simulink model "BalRobModel"  (R2021a)
settings: Solver=FixedStepAuto  StartTime=0.0  StopTime=20  FixedStep=Ts  RelTol=1e-3
undefined symbols (not defined in the file): body, DiscIntNeverNeededParam, drv, g, gbox, lqr_nominal, lqr_robust, mot, ms22g, nlmodel, Nu, Nx, sens, stvar_est, Ts, wheel
settings Model: Creator=gioel  LastModifiedBy=gioel
settings DataIOCC: LimitDataPoints=on  MaxDataPoints=50000  ReturnWorkspaceOutputs=off
settings DebuggingCC: AlgebraicLoopMsg=none

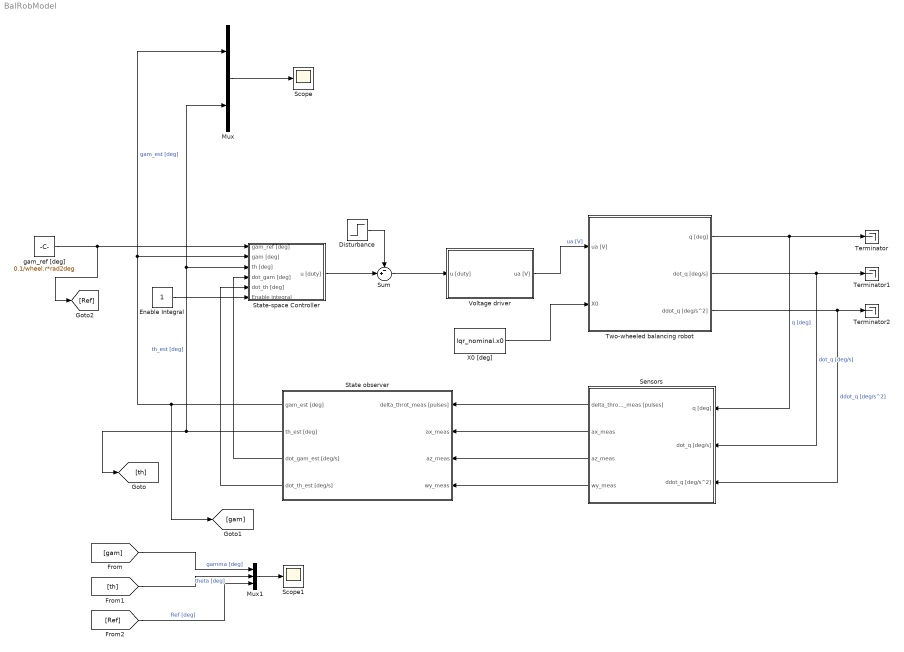
== system BalRobModel ==
  Disturbance : Step  Time=10  After=5/drv.duty2V  SampleTime=0
  Enable Integral : Constant
  Mux : Mux  Inputs=2
  Mux1 : Mux  Inputs=3
  Scope : Scope
  Scope1 : Scope
  Sensors : Subsystem
  State observer : Subsystem
  State-space Controller : Subsystem
  Sum : Sum  Inputs=-+|
  Terminator : Terminator
  Terminator1 : Terminator
  Terminator2 : Terminator
  Two-wheeled balancing robot : Subsystem
  Voltage driver : Subsystem
  X0 [deg] : Constant  Value=lqr_nominal.x0
  gam_ref [deg] : Constant  Value=0.1/wheel.r*rad2deg
  wires:
  Voltage driver/1(ua [V]) -> Two-wheeled balancing robot/1(ua [V])  "ua [V]"
  Two-wheeled balancing robot/1(q [deg]) -> Sensors/1(q [deg]), Terminator/1  "q [deg]"
  Two-wheeled balancing robot/2(dot_q [deg/s]) -> Sensors/2(dot_q [deg/s]), Terminator1/1  "dot_q [deg/s]"
  Two-wheeled balancing robot/3(ddot_q [deg/s^2]) -> Sensors/3(ddot_q [deg/s^2]), Terminator2/1  "ddot_q [deg/s^2]"
  State observer/2(th_est [deg]) -> [th], Mux/2, State-space Controller/3(th [deg])  "th_est [deg]"
  State observer/1(gam_est [deg]) -> [gam], Mux/1, State-space Controller/2(gam [deg])  "gam_est [deg]"
  State observer/3(dot_gam_est [deg/s]) -> State-space Controller/4(dot_gam [deg])
  Sensors/1(delta_throt_meas [pulses]) -> State observer/1(delta_throt_meas [pulses])
  Sensors/2(ax_meas) -> State observer/2(ax_meas)
  Sensors/3(az_meas) -> State observer/3(az_meas)
  Sensors/4(wy_meas) -> State observer/4(wy_meas)
  gam_ref [deg]/1 -> [Ref], State-space Controller/1(gam_ref [deg])
  State observer/4(dot_th_est [deg/s]) -> State-space Controller/5(dot_th [deg])
  Mux/1 -> Scope/1
  Enable Integral/1 -> State-space Controller/6(Enable integral)
  State-space Controller/1(u [duty]) -> Sum/2
  Sum/1 -> Voltage driver/1(u [duty])
  Disturbance/1 -> Sum/1
  X0 [deg]/1 -> Two-wheeled balancing robot/2(X0)
  [gam] -> Mux1/1  "gamma [deg]"
  [th] -> Mux1/2  "theta [deg]"
  Mux1/1 -> Scope1/1
  [Ref] -> Mux1/3  "Ref [deg]"

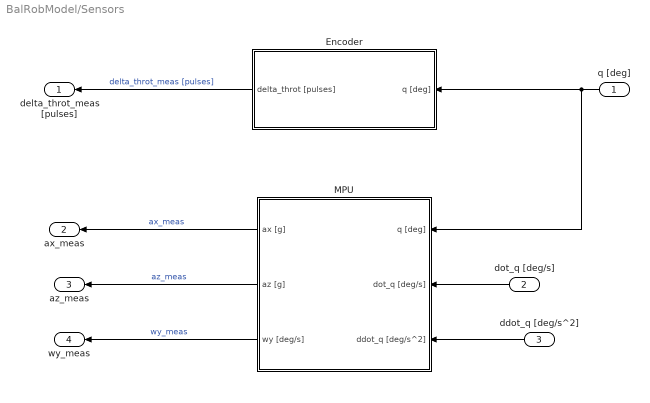
== system BalRobModel/Sensors ==
  q [deg] : Inport
  dot_q [deg/s] : Inport  Port=2
  ddot_q [deg/s^2] : Inport  Port=3
  Encoder : Subsystem
  MPU : Subsystem
  delta_throt_meas [pulses] : Outport
  ax_meas : Outport  Port=2
  az_meas : Outport  Port=3
  wy_meas : Outport  Port=4
  wires:
  Encoder/1(delta_throt [pulses]) -> delta_throt_meas [pulses]/1  "delta_throt_meas [pulses]"
  MPU/3(wy [deg/s]) -> wy_meas/1  "wy_meas"
  ddot_q [deg/s^2]/1 -> MPU/3(ddot_q [deg/s^2])
  MPU/2(az [g]) -> az_meas/1  "az_meas"
  dot_q [deg/s]/1 -> MPU/2(dot_q [deg/s])
  MPU/1(ax [g]) -> ax_meas/1  "ax_meas"
  q [deg]/1 -> MPU/1(q [deg]), Encoder/1(q [deg])

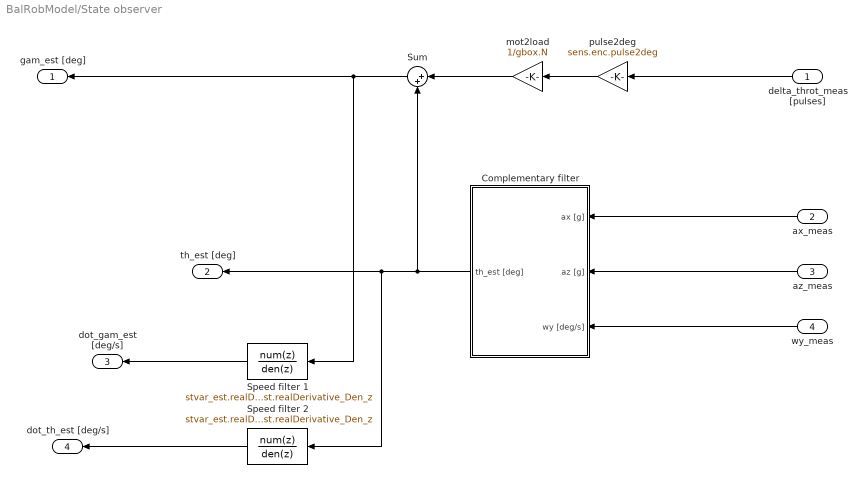
== system BalRobModel/State observer ==
  delta_throt_meas [pulses] : Inport
  ax_meas : Inport  Port=2
  az_meas : Inport  Port=3
  wy_meas : Inport  Port=4
  Complementary filter : Subsystem
  Speed filter 1 : DiscreteTransferFcn  Numerator=stvar_est.realDerivative_Num_z  Denominator=stvar_est.realDerivative_Den_z  SampleTime=Ts
  Speed filter 2 : DiscreteTransferFcn  Numerator=stvar_est.realDerivative_Num_z  Denominator=stvar_est.realDerivative_Den_z  SampleTime=Ts
  Sum : Sum  Inputs=|++
  mot2load : Gain  Gain=1/gbox.N
  pulse2deg : Gain  Gain=sens.enc.pulse2deg
  gam_est [deg] : Outport
  th_est [deg] : Outport  Port=2
  dot_gam_est [deg/s] : Outport  Port=3
  dot_th_est [deg/s] : Outport  Port=4
  wires:
  az_meas/1 -> Complementary filter/2(az [g])
  Speed filter 1/1 -> dot_gam_est [deg/s]/1
  Speed filter 2/1 -> dot_th_est [deg/s]/1
  wy_meas/1 -> Complementary filter/3(wy [deg/s])
  ax_meas/1 -> Complementary filter/1(ax [g])
  delta_throt_meas [pulses]/1 -> pulse2deg/1
  pulse2deg/1 -> mot2load/1
  mot2load/1 -> Sum/1
  Sum/1 -> gam_est [deg]/1, Speed filter 1/1
  Complementary filter/1(th_est [deg]) -> Sum/2, th_est [deg]/1, Speed filter 2/1

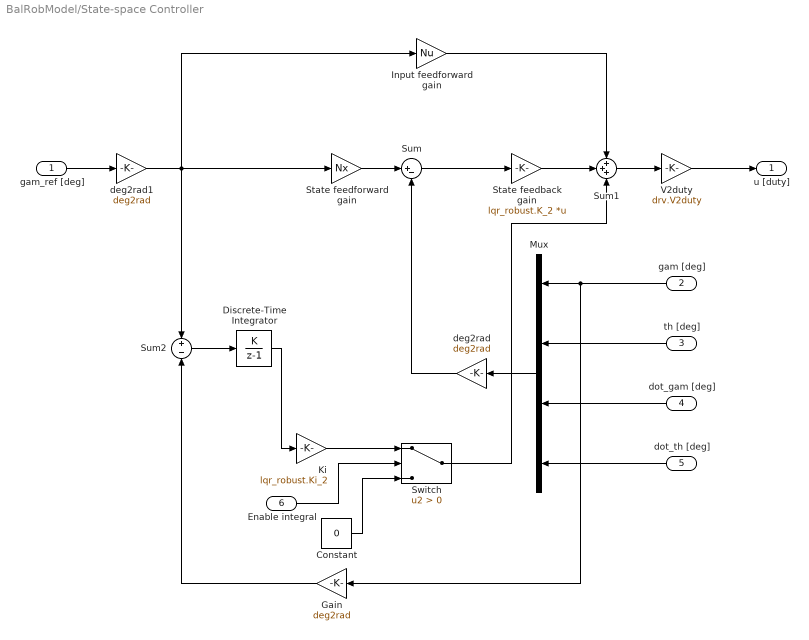
== system BalRobModel/State-space Controller ==
  gam_ref [deg] : Inport
  gam [deg] : Inport  Port=2
  th [deg] : Inport  Port=3
  dot_gam [deg] : Inport  Port=4
  dot_th [deg] : Inport  Port=5
  Enable integral : Inport  Port=6
  Constant : Constant  Value=0
  Discrete-Time Integrator : DiscreteIntegrator  IntegratorMethod=Accumulation: Forward Euler  SampleTime=Ts  ICPrevOutput=DiscIntNeverNeededParam  ICPrevScaledInput=DiscIntNeverNeededParam
  Gain : Gain  Gain=deg2rad
  Input feedforward gain : Gain  Gain=Nu
  Ki : Gain  Gain=lqr_robust.Ki_2
  Mux : Mux
  State feedback gain : Gain  Gain=lqr_robust.K_2  Multiplication=Matrix(K*u)
  State feedforward gain : Gain  Gain=Nx
  Sum : Sum  Inputs=|+-
  Sum1 : Sum  Inputs=+++
  Sum2 : Sum  Inputs=+|-
  Switch : Switch  Criteria=u2 > Threshold
  V2duty : Gain  Gain=drv.V2duty
  deg2rad : Gain  Gain=deg2rad
  deg2rad1 : Gain  Gain=deg2rad
  u [duty] : Outport
  wires:
  gam [deg]/1 -> Gain/1, Mux/1
  th [deg]/1 -> Mux/2
  dot_gam [deg]/1 -> Mux/3
  dot_th [deg]/1 -> Mux/4
  Mux/1 -> deg2rad/1
  gam_ref [deg]/1 -> deg2rad1/1
  deg2rad1/1 -> State feedforward gain/1, Input feedforward gain/1, Sum2/1
  State feedforward gain/1 -> Sum/1
  deg2rad/1 -> Sum/2
  Sum/1 -> State feedback gain/1
  State feedback gain/1 -> Sum1/2
  Input feedforward gain/1 -> Sum1/1
  Sum1/1 -> V2duty/1
  V2duty/1 -> u [duty]/1
  Gain/1 -> Sum2/2
  Sum2/1 -> Discrete-Time Integrator/1
  Discrete-Time Integrator/1 -> Ki/1
  Ki/1 -> Switch/1
  Switch/1 -> Sum1/3
  Enable integral/1 -> Switch/2
  Constant/1 -> Switch/3

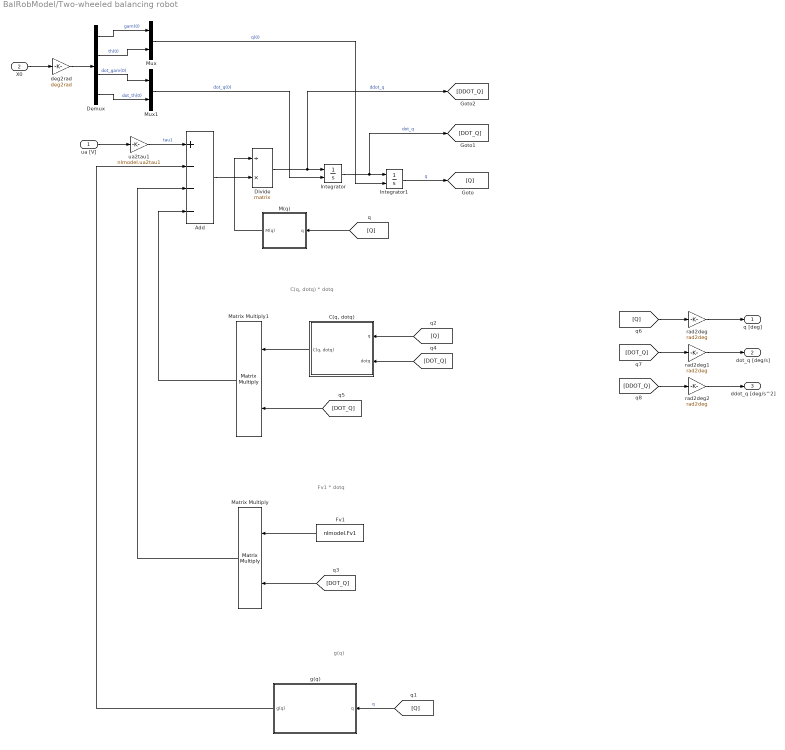
== system BalRobModel/Two-wheeled balancing robot ==
  note: g(q)
  note: Fv1 * dotq
  note: C(q, dotq) * dotq
  ua [V] : Inport
  X0 : Inport  Port=2
  Add : Sum  Inputs=+---
  "C(q, dotq)" : Subsystem
  Demux : Demux
  Divide : Product  Inputs=/*  Multiplication=Matrix(*)
  Fv1 : Constant  Value=nlmodel.Fv1
  Integrator : Integrator  InitialConditionSource=external  InitialCondition=[0;0]
  Integrator1 : Integrator  InitialConditionSource=external  InitialCondition=[0; 0]
  M(q) : Subsystem
  Matrix Multiply : Product  Multiplication=Matrix(*)
  Matrix Multiply1 : Product  Multiplication=Matrix(*)
  Mux : Mux  Inputs=2
  Mux1 : Mux  Inputs=2
  deg2rad : Gain  Gain=deg2rad
  g(q) : Subsystem
  rad2deg : Gain  Gain=rad2deg
  rad2deg1 : Gain  Gain=rad2deg
  rad2deg2 : Gain  Gain=rad2deg
  ua2tau1 : Gain  Gain=nlmodel.ua2tau1
  q [deg] : Outport
  dot_q [deg/s] : Outport  Port=2
  ddot_q [deg/s^2] : Outport  Port=3
  wires:
  [Q] -> M(q)/1(q)
  [Q] -> g(q)/1(q)  "q"
  [DOT_Q] -> rad2deg1/1
  rad2deg1/1 -> dot_q [deg/s]/1
  Matrix Multiply/1 -> Add/3
  Add/1 -> Divide/2
  Divide/1 -> [DDOT_Q], Integrator/1  "ddot_q"
  "C(q, dotq)"/1("C(q, dotq)") -> Matrix Multiply1/1
  rad2deg2/1 -> ddot_q [deg/s^2]/1
  g(q)/1(g(q)) -> Add/2
  M(q)/1(M(q)) -> Divide/1
  [Q] -> rad2deg/1
  [DDOT_Q] -> rad2deg2/1
  ua [V]/1 -> ua2tau1/1
  [Q] -> "C(q, dotq)"/1(q)
  Integrator/1 -> Integrator1/1, [DOT_Q]  "dot_q"
  ua2tau1/1 -> Add/1  "tau1"
  [DOT_Q] -> "C(q, dotq)"/2(dotq)
  [DOT_Q] -> Matrix Multiply/2
  [DOT_Q] -> Matrix Multiply1/2
  Integrator1/1 -> [Q]  "q"
  Matrix Multiply1/1 -> Add/4
  rad2deg/1 -> q [deg]/1
  Fv1/1 -> Matrix Multiply/1
  Demux/1 -> Mux/1  "gam(0)"
  Demux/2 -> Mux/2  "th(0)"
  Demux/3 -> Mux1/1  "dot_gam(0)"
  Demux/4 -> Mux1/2  "dot_th(0)"
  X0/1 -> deg2rad/1
  deg2rad/1 -> Demux/1
  Mux/1 -> Integrator1/2  "q(0)"
  Mux1/1 -> Integrator/2  "dot_q(0)"

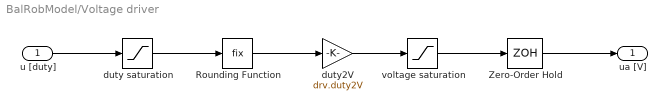
== system BalRobModel/Voltage driver ==
  u [duty] : Inport
  Rounding Function : Rounding  Operator=fix
  Zero-Order Hold : ZeroOrderHold  SampleTime=Ts
  duty saturation : Saturate  UpperLimit=drv.dutymax  LowerLimit=-drv.dutymax
  duty2V : Gain  Gain=drv.duty2V
  voltage saturation : Saturate  UpperLimit=drv.Vbus  LowerLimit=-drv.Vbus
  ua [V] : Outport
  wires:
  u [duty]/1 -> duty saturation/1
  duty saturation/1 -> Rounding Function/1
  Rounding Function/1 -> duty2V/1
  duty2V/1 -> voltage saturation/1
  voltage saturation/1 -> Zero-Order Hold/1
  Zero-Order Hold/1 -> ua [V]/1

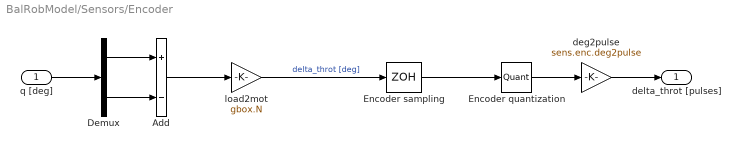
== system BalRobModel/Sensors/Encoder ==
  q [deg] : Inport
  Add : Sum  Inputs=+-
  Demux : Demux  Outputs=2
  Encoder quantization : Quantizer  QuantizationInterval=sens.enc.pulse2deg
  Encoder sampling : ZeroOrderHold  SampleTime=Ts
  deg2pulse : Gain  Gain=sens.enc.deg2pulse
  load2mot : Gain  Gain=gbox.N
  delta_throt [pulses] : Outport
  wires:
  q [deg]/1 -> Demux/1
  Demux/2 -> Add/2
  Demux/1 -> Add/1
  Add/1 -> load2mot/1
  load2mot/1 -> Encoder sampling/1  "delta_throt [deg]"
  Encoder sampling/1 -> Encoder quantization/1
  deg2pulse/1 -> delta_throt [pulses]/1
  Encoder quantization/1 -> deg2pulse/1

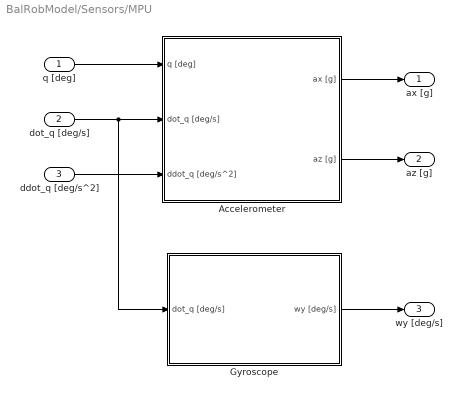
== system BalRobModel/Sensors/MPU ==
  q [deg] : Inport
  dot_q [deg/s] : Inport  Port=2
  ddot_q [deg/s^2] : Inport  Port=3
  "\tGyroscope" : Subsystem
  Accelerometer : Subsystem
  ax [g] : Outport
  az [g] : Outport  Port=2
  wy [deg/s] : Outport  Port=3
  wires:
  ddot_q [deg/s^2]/1 -> Accelerometer/3(ddot_q [deg/s^2])
  dot_q [deg/s]/1 -> "\tGyroscope"/1(dot_q [deg/s]), Accelerometer/2(dot_q [deg/s])
  q [deg]/1 -> Accelerometer/1(q [deg])
  "\tGyroscope"/1(wy [deg/s]) -> wy [deg/s]/1
  Accelerometer/2(az [g]) -> az [g]/1
  Accelerometer/1(ax [g]) -> ax [g]/1

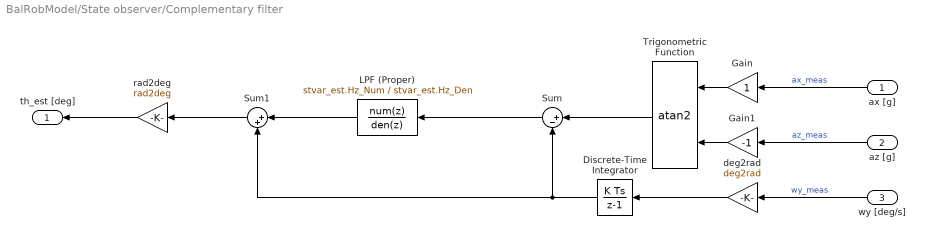
== system BalRobModel/State observer/Complementary filter ==
  ax [g] : Inport
  az [g] : Inport  Port=2
  wy [deg/s] : Inport  Port=3
  Discrete-Time Integrator : DiscreteIntegrator  SampleTime=Ts  ICPrevOutput=DiscIntNeverNeededParam  ICPrevScaledInput=DiscIntNeverNeededParam
  Gain : Gain
  Gain1 : Gain  Gain=-1
  LPF (Proper) : DiscreteTransferFcn  Numerator=stvar_est.Hz_Num  Denominator=stvar_est.Hz_Den  SampleTime=Ts
  Sum : Sum  Inputs=|+-
  Sum1 : Sum  Inputs=|++
  Trigonometric Function : Trigonometry  Operator=atan2
  deg2rad : Gain  Gain=deg2rad
  rad2deg : Gain  Gain=rad2deg
  th_est [deg] : Outport
  wires:
  LPF (Proper)/1 -> Sum1/1
  rad2deg/1 -> th_est [deg]/1
  Sum/1 -> LPF (Proper)/1
  Sum1/1 -> rad2deg/1
  Discrete-Time Integrator/1 -> Sum1/2, Sum/2
  Trigonometric Function/1 -> Sum/1
  wy [deg/s]/1 -> deg2rad/1  "wy_meas"
  az [g]/1 -> Gain1/1  "az_meas"
  ax [g]/1 -> Gain/1  "ax_meas"
  deg2rad/1 -> Discrete-Time Integrator/1
  Gain1/1 -> Trigonometric Function/2
  Gain/1 -> Trigonometric Function/1

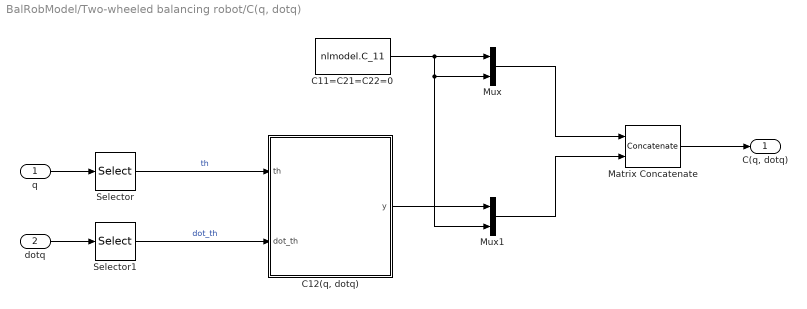
== system BalRobModel/Two-wheeled balancing robot/C(q, dotq) ==
  q : Inport
  dotq : Inport  Port=2
  C11=C21=C22=0 : Constant  Value=nlmodel.C_11
  "C12(q, dotq)" : MATLAB Function  TreatAsAtomicUnit=on
  Matrix Concatenate : Concatenate  Mode=Multidimensional array  ConcatenateDimension=2
  Mux : Mux  Inputs=2
  Mux1 : Mux  Inputs=2
  Selector : Selector  InputPortWidth=2  IndexOptions=Starting index (dialog)  Indices=2  OutputSizes=1
  Selector1 : Selector  InputPortWidth=2  IndexOptions=Starting index (dialog)  Indices=2  OutputSizes=1
  "C(q, dotq)" : Outport
  wires:
  Matrix Concatenate/1 -> "C(q, dotq)"/1
  "C12(q, dotq)"/1(y) -> Mux1/1
  q/1 -> Selector/1
  dotq/1 -> Selector1/1
  Selector1/1 -> "C12(q, dotq)"/2(dot_th)  "dot_th"
  Selector/1 -> "C12(q, dotq)"/1(th)  "th"
  C11=C21=C22=0/1 -> Mux/2, Mux1/2, Mux/1
  Mux/1 -> Matrix Concatenate/1
  Mux1/1 -> Matrix Concatenate/2

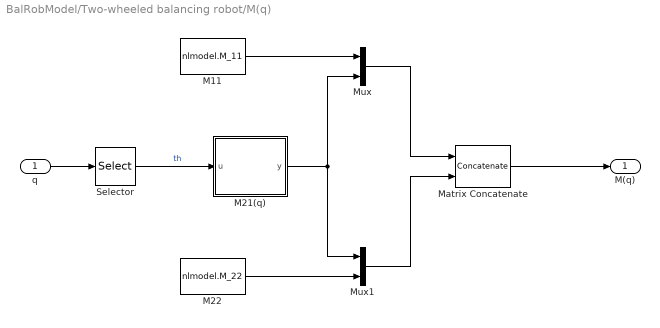
== system BalRobModel/Two-wheeled balancing robot/M(q) ==
  q : Inport
  M11 : Constant  Value=nlmodel.M_11
  M21(q) : MATLAB Function  TreatAsAtomicUnit=on
  M22 : Constant  Value=nlmodel.M_22
  Matrix Concatenate : Concatenate  Mode=Multidimensional array  ConcatenateDimension=2
  Mux : Mux  Inputs=2
  Mux1 : Mux  Inputs=2
  Selector : Selector  InputPortWidth=2  IndexOptions=Starting index (dialog)  Indices=2  OutputSizes=1
  M(q) : Outport
  wires:
  Matrix Concatenate/1 -> M(q)/1
  Mux1/1 -> Matrix Concatenate/2
  M22/1 -> Mux1/2
  M11/1 -> Mux/1
  Selector/1 -> M21(q)/1(u)  "th"
  M21(q)/1(y) -> Mux1/1, Mux/2
  q/1 -> Selector/1
  Mux/1 -> Matrix Concatenate/1

== system BalRobModel/Two-wheeled balancing robot/g(q) ==
  q : Inport
  Mux : Mux  Inputs=2
  Selector : Selector  InputPortWidth=2  IndexOptions=Starting index (dialog)  Indices=2  OutputSizes=1
  g1 : Constant  Value=nlmodel.g_1
  g2(q) : MATLAB Function  TreatAsAtomicUnit=on
  g(q) : Outport
  wires:
  g2(q)/1(y) -> Mux/2
  q/1 -> Selector/1
  Selector/1 -> g2(q)/1(u)  "th"
  Mux/1 -> g(q)/1
  g1/1 -> Mux/1

== system BalRobModel/Sensors/MPU/	Gyroscope ==
  dot_q [deg/s] : Inport
  Random Number : RandomNumber  Variance=sens.mpu.gyro.noisevar  SampleTime=Ts
  Selector : Selector  InputPortWidth=2  IndexOptions=Starting index (dialog)  Indices=2  OutputSizes=1
  Sum : Sum  Inputs=++|
  y-axis quantization : Quantizer  QuantizationInterval=sens.mpu.gyro.LSB2degs
  y-axis sampling : ZeroOrderHold  SampleTime=Ts
  wy [deg/s] : Outport
  wires:
  dot_q [deg/s]/1 -> Selector/1
  Selector/1 -> y-axis sampling/1  "dot_th"
  y-axis sampling/1 -> Sum/2
  Random Number/1 -> Sum/1
  Sum/1 -> y-axis quantization/1
  y-axis quantization/1 -> wy [deg/s]/1

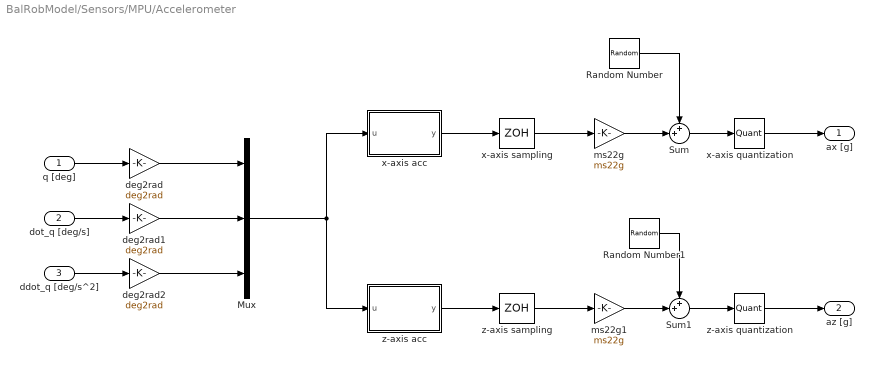
== system BalRobModel/Sensors/MPU/Accelerometer ==
  q [deg] : Inport
  dot_q [deg/s] : Inport  Port=2
  ddot_q [deg/s^2] : Inport  Port=3
  Mux : Mux  Inputs=3
  Random Number : RandomNumber  Variance=sens.mpu.acc.noisevar  SampleTime=Ts
  Random Number1 : RandomNumber  Variance=sens.mpu.acc.noisevar  SampleTime=Ts
  Sum : Sum  Inputs=++|
  Sum1 : Sum  Inputs=++|
  deg2rad : Gain  Gain=deg2rad
  deg2rad1 : Gain  Gain=deg2rad
  deg2rad2 : Gain  Gain=deg2rad
  ms22g : Gain  Gain=ms22g
  ms22g1 : Gain  Gain=ms22g
  x-axis acc : MATLAB Function  TreatAsAtomicUnit=on
  x-axis quantization : Quantizer  QuantizationInterval=sens.mpu.acc.LSB2g
  x-axis sampling : ZeroOrderHold  SampleTime=Ts
  z-axis acc : MATLAB Function  TreatAsAtomicUnit=on
  z-axis quantization : Quantizer  QuantizationInterval=sens.mpu.acc.LSB2g
  z-axis sampling : ZeroOrderHold  SampleTime=Ts
  ax [g] : Outport
  az [g] : Outport  Port=2
  wires:
  q [deg]/1 -> deg2rad/1
  ddot_q [deg/s^2]/1 -> deg2rad2/1
  dot_q [deg/s]/1 -> deg2rad1/1
  deg2rad/1 -> Mux/1
  deg2rad2/1 -> Mux/3
  deg2rad1/1 -> Mux/2
  Mux/1 -> z-axis acc/1(u), x-axis acc/1(u)
  x-axis acc/1(y) -> x-axis sampling/1
  z-axis acc/1(y) -> z-axis sampling/1
  x-axis sampling/1 -> ms22g/1
  z-axis sampling/1 -> ms22g1/1
  ms22g/1 -> Sum/2
  ms22g1/1 -> Sum1/2
  Random Number/1 -> Sum/1
  Random Number1/1 -> Sum1/1
  Sum/1 -> x-axis quantization/1
  Sum1/1 -> z-axis quantization/1
  x-axis quantization/1 -> ax [g]/1
  z-axis quantization/1 -> az [g]/1

== matlab function BalRobModel/Two-wheeled balancing robot/g(q)/g2(q) ==
  data: u input; y output; mot parameter; body parameter; g parameter
function y = f(u, mot, body, g)
y = -(body.m * body.zb + 2 * mot.rot.m * mot.rot.zb) * g * sin(u);

== matlab function BalRobModel/Two-wheeled balancing robot/C(q, dotq)/C12(q, dotq) ==
  data: th input; y output; dot_th input; mot parameter; wheel parameter; body parameter
function y = f(th, dot_th, mot, wheel, body)
y = -(body.m * body.zb + 2 * mot.rot.m * mot.rot.zb) * wheel.r * sin(th) * dot_th;

== matlab function BalRobModel/Two-wheeled balancing robot/M(q)/M21(q) ==
  data: u input; y output; gbox parameter; mot parameter; body parameter; wheel parameter
function y = f(u, gbox, mot, body, wheel)
y = 2 * gbox.N * (1-gbox.N) * mot.rot.Iyy + (body.m * body.zb + 2 * mot.rot.m * mot.rot.zb) * wheel.r * cos(u);

== matlab function BalRobModel/Sensors/MPU/Accelerometer/x-axis acc ==
  data: u input; y output; wheel parameter; sens parameter; g parameter
function y = fcn(u, wheel, sens, g)
y = wheel.r*u(5)*cos(u(2)) + sens.mpu.zb*u(6) + g*sin(u(2));

== matlab function BalRobModel/Sensors/MPU/Accelerometer/z-axis acc ==
  data: u input; y output; wheel parameter; sens parameter; g parameter
function y = fcn(u, wheel, sens, g)
y = wheel.r*u(5)*sin(u(2)) - sens.mpu.zb*u(4)^2 - g*cos(u(2));
